simulink library "inp"  (R2021b)
settings: Solver=VariableStepAuto  StartTime=0.0  StopTime=10.0  RelTol=1e-3
undefined symbols (not defined in the file): C_TASK_5MS_S, FALSE, KINP_AcoreReadyToSlp_flg_ovrdflg, KINP_AcoreReadyToSlp_flg_ovrdval, KINP_AllowMovThd_OTA_enum_ovrdflg, KINP_AllowMovThd_OTA_enum_ovrdval, KINP_APSAngleTarget_Deg_ovrdflg, KINP_APSAngleTarget_Deg_ovrdval, KINP_APSDecReq_mps2_ovrdflg, KINP_APSDecReq_mps2_ovrdval, KINP_APSDecReqA_flg_ovrdflg, KINP_APSDecReqA_flg_ovrdval, KINP_APSDFLL_cm_ovrdflg, KINP_APSDFLL_cm_ovrdval, KINP_APSDFLR_cm_ovrdflg, KINP_APSDFLR_cm_ovrdval, KINP_APSDRLL_cm_ovrdflg, KINP_APSDRLL_cm_ovrdval, KINP_APSDRLR_cm_ovrdflg, KINP_APSDRLR_cm_ovrdval, KINP_APSExitCondition_enum_ovrdflg, KINP_APSExitCondition_enum_ovrdval, KINP_APSHWVer_enum_ovrdflg, KINP_APSHWVer_enum_ovrdval, KINP_APSProgressPCT_pct_ovrdflg, KINP_APSProgressPCT_pct_ovrdval, KINP_APSReq_enum_ovrdflg, KINP_APSReq_enum_ovrdval, KINP_APSRQDisplay_enum_ovrdflg, KINP_APSRQDisplay_enum_ovrdval, KINP_APSRqEPASCtrl_flg_ovrdflg, KINP_APSRqEPASCtrl_flg_ovrdval, KINP_APSShiftPosnReq_enum_ovrdval, KINP_APSShiftPosnReq_enum_ovrflg, KINP_APSSpeedCMD_kph_ovrdval, KINP_APSSpeedCMD_kph_ovrflg, KINP_APSStaSystem_enum_ovrdflg, KINP_APSStaSystem_enum_ovrdval, KINP_APSSWVer_enum_ovrdflg, KINP_APSSWVer_enum_ovrdval, KINP_APSVMCReqA_flg_ovrdval, KINP_APSVMCReqA_flg_ovrflg, KINP_APSVRqEPASCtrl_flg_ovrdflg, KINP_APSVRqEPASCtrl_flg_ovrdval, KINP_AuxBattVolmV_mV_ovrdflg, KINP_AuxBattVolmV_mV_ovrdval, KINP_CAASSta_enum_ovrdflg, KINP_CAASSta_enum_ovrdval, KINP_CAASVMCReqA_flg_ovrdval, KINP_CAASVMCReqA_flg_ovrflg, KINP_Chime_enum_ovrdflg, KINP_Chime_enum_ovrdval, KINP_ClearDTCcmd_flg_ovrdflg, KINP_ClearDTCcmd_flg_ovrdval, KINP_EvccAplusPwrUpReq_flg_ovrdflg, KINP_EvccAplusPwrUpReq_flg_ovrdval, KINP_LFID_raw_ovrdval, KINP_LFID_raw_ovrflg, KINP_LRID_raw_ovrdval, KINP_MemOffsetAccX_raw16_ovrdflg ... (+118)
libraries: FVT_lib x595, hcu_lib x1
(part 9 of 27)

== system inp/INP/CAN1/SignalCheck/EPAS2 ==
  BHAL_outputs : Inport
  inp_CanValid_bus : Inport  Port=2
  SASAngle : FVT_lib/inp/can_signal_template  SystemSampleTime=-1  VariantActivationTime=update diagram  Latency=0  AutoFrameSizeCalculation=off
      link override defval: Value=KINP_SASAngle_Deg_defval
      link override fftdec: Value=KINP_SASAngle_Deg_fftdec
      link override fftinc: Value=KINP_SASAngle_Deg_fftinc
      link override fftlim: Value=KINP_SASAngle_Deg_fftlim
      link override invalid: Value=KINP_SASAngle_Deg_invalid
      link override ovrdflg: Value=KINP_SASAngle_Deg_ovrdflg
      link override ovrdval: Value=KINP_SASAngle_Deg_ovrdval
      link override setvalid: Value=KINP_SASAngle_Deg_setvalid
      link override srvcflg: Value=KINP_SASAngle_Deg_srvcflg
      link override srvcval: Value=KINP_SASAngle_Deg_srvcval
  SASCAL : FVT_lib/inp/can_signal_template  SystemSampleTime=-1  VariantActivationTime=update diagram  Latency=0  AutoFrameSizeCalculation=off
      link override defval: Value=KINP_SASCAL_flg_defval
      link override fftdec: Value=KINP_SASCAL_flg_fftdec
      link override fftinc: Value=KINP_SASCAL_flg_fftinc
      link override fftlim: Value=KINP_SASCAL_flg_fftlim
      link override invalid: Value=KINP_SASCAL_flg_invalid
      link override ovrdflg: Value=KINP_SASCAL_flg_ovrdflg
      link override ovrdval: Value=KINP_SASCAL_flg_ovrdval
      link override setvalid: Value=KINP_SASCAL_flg_setvalid
      link override srvcflg: Value=KINP_SASCAL_flg_srvcflg
      link override srvcval: Value=KINP_SASCAL_flg_srvcval
  SASSpeed : FVT_lib/inp/can_signal_template  SystemSampleTime=-1  VariantActivationTime=update diagram  Latency=0  AutoFrameSizeCalculation=off
      link override defval: Value=KINP_SASSpeed_degps_defval
      link override fftdec: Value=KINP_SASSpeed_degps_fftdec
      link override fftinc: Value=KINP_SASSpeed_degps_fftinc
      link override fftlim: Value=KINP_SASSpeed_degps_fftlim
      link override invalid: Value=KINP_SASSpeed_degps_invalid
      link override ovrdflg: Value=KINP_SASSpeed_degps_ovrdflg
      link override ovrdval: Value=KINP_SASSpeed_degps_ovrdval
      link override setvalid: Value=KINP_SASSpeed_degps_setvalid
      link override srvcflg: Value=KINP_SASSpeed_degps_srvcflg
      link override srvcval: Value=KINP_SASSpeed_degps_srvcval
  SASSpeedValid : FVT_lib/inp/can_signal_template  SystemSampleTime=-1  VariantActivationTime=update diagram  Latency=0  AutoFrameSizeCalculation=off
      link override defval: Value=KINP_SASSpeedValid_flg_defval
      link override fftdec: Value=KINP_SASSpeedValid_flg_fftdec
      link override fftinc: Value=KINP_SASSpeedValid_flg_fftinc
      link override fftlim: Value=KINP_SASSpeedValid_flg_fftlim
      link override invalid: Value=KINP_SASSpeedValid_flg_invalid
      link override ovrdflg: Value=KINP_SASSpeedValid_flg_ovrdflg
      link override ovrdval: Value=KINP_SASSpeedValid_flg_ovrdval
      link override setvalid: Value=KINP_SASSpeedValid_flg_setvalid
      link override srvcflg: Value=KINP_SASSpeedValid_flg_srvcflg
      link override srvcval: Value=KINP_SASSpeedValid_flg_srvcval
  SASV : FVT_lib/inp/can_signal_template  SystemSampleTime=-1  VariantActivationTime=update diagram  Latency=0  AutoFrameSizeCalculation=off
      link override defval: Value=KINP_SASV_flg_defval
      link override fftdec: Value=KINP_SASV_flg_fftdec
      link override fftinc: Value=KINP_SASV_flg_fftinc
      link override fftlim: Value=KINP_SASV_flg_fftlim
      link override invalid: Value=KINP_SASV_flg_invalid
      link override ovrdflg: Value=KINP_SASV_flg_ovrdflg
      link override ovrdval: Value=KINP_SASV_flg_ovrdval
      link override setvalid: Value=KINP_SASV_flg_setvalid
      link override srvcflg: Value=KINP_SASV_flg_srvcflg
      link override srvcval: Value=KINP_SASV_flg_srvcval
  Terminator_{1..5} (5 alike) : Terminator
  True_VHAL_SASAngle_Deg : Constant  Value=TRUE  OutDataTypeStr=boolean
  True_VHAL_SASCAL_flg : Constant  Value=TRUE  OutDataTypeStr=boolean
  True_VHAL_SASSpeedValid_flg : Constant  Value=TRUE  OutDataTypeStr=boolean
  True_VHAL_SASSpeed_degps : Constant  Value=TRUE  OutDataTypeStr=boolean
  True_VHAL_SASV_flg : Constant  Value=TRUE  OutDataTypeStr=boolean
  slr1_{1..5} (5 alike) : BusSelector  OutputSignals=VINP_CANMsgValidEPAS2_flg
  slr_VHAL_SASAngle_Deg : BusSelector  OutputSignals=VHAL_SASAngle_Deg
  slr_VHAL_SASCAL_flg : BusSelector  OutputSignals=VHAL_SASCAL_flg
  slr_VHAL_SASSpeedValid_flg : BusSelector  OutputSignals=VHAL_SASSpeedValid_flg
  slr_VHAL_SASSpeed_degps : BusSelector  OutputSignals=VHAL_SASSpeed_degps
  slr_VHAL_SASV_flg : BusSelector  OutputSignals=VHAL_SASV_flg
  VINP_SASAngle_Deg : Outport
  VINP_SASCAL_flg : Outport  Port=2
  VINP_SASSpeed_degps : Outport  Port=3
  VINP_SASSpeedValid_flg : Outport  Port=4
  VINP_SASV_flg : Outport  Port=5
  wires:
  BHAL_outputs/1 -> [BHAL_outputs]
  inp_CanValid_bus/1 -> [inp_CanValid_bus]
  [BHAL_outputs] -> slr_VHAL_SASAngle_Deg/1
  slr_VHAL_SASAngle_Deg/1 -> SASAngle/1  "<VHAL_SASAngle_Deg>"
  True_VHAL_SASAngle_Deg/1 -> SASAngle/2
  [inp_CanValid_bus] -> slr1_1/1
  slr1_1/1 -> SASAngle/3  "<VINP_CANMsgValidEPAS2_flg>"
  SASAngle/1 -> VINP_SASAngle_Deg/1  "VINP_SASAngle_Deg"
  SASAngle/2 -> Terminator_1/1
  [BHAL_outputs] -> slr_VHAL_SASCAL_flg/1
  slr_VHAL_SASCAL_flg/1 -> SASCAL/1  "<VHAL_SASCAL_flg>"
  True_VHAL_SASCAL_flg/1 -> SASCAL/2
  [inp_CanValid_bus] -> slr1_2/1
  slr1_2/1 -> SASCAL/3  "<VINP_CANMsgValidEPAS2_flg>"
  SASCAL/1 -> VINP_SASCAL_flg/1  "VINP_SASCAL_flg"
  SASCAL/2 -> Terminator_2/1
  [BHAL_outputs] -> slr_VHAL_SASSpeed_degps/1
  slr_VHAL_SASSpeed_degps/1 -> SASSpeed/1  "<VHAL_SASSpeed_degps>"
  True_VHAL_SASSpeed_degps/1 -> SASSpeed/2
  [inp_CanValid_bus] -> slr1_3/1
  slr1_3/1 -> SASSpeed/3  "<VINP_CANMsgValidEPAS2_flg>"
  SASSpeed/1 -> VINP_SASSpeed_degps/1  "VINP_SASSpeed_degps"
  SASSpeed/2 -> Terminator_3/1
  [BHAL_outputs] -> slr_VHAL_SASSpeedValid_flg/1
  slr_VHAL_SASSpeedValid_flg/1 -> SASSpeedValid/1  "<VHAL_SASSpeedValid_flg>"
  True_VHAL_SASSpeedValid_flg/1 -> SASSpeedValid/2
  [inp_CanValid_bus] -> slr1_4/1
  slr1_4/1 -> SASSpeedValid/3  "<VINP_CANMsgValidEPAS2_flg>"
  SASSpeedValid/1 -> VINP_SASSpeedValid_flg/1  "VINP_SASSpeedValid_flg"
  SASSpeedValid/2 -> Terminator_4/1
  [BHAL_outputs] -> slr_VHAL_SASV_flg/1
  slr_VHAL_SASV_flg/1 -> SASV/1  "<VHAL_SASV_flg>"
  True_VHAL_SASV_flg/1 -> SASV/2
  [inp_CanValid_bus] -> slr1_5/1
  slr1_5/1 -> SASV/3  "<VINP_CANMsgValidEPAS2_flg>"
  SASV/1 -> VINP_SASV_flg/1  "VINP_SASV_flg"
  SASV/2 -> Terminator_5/1

== system inp/INP/CAN1/SignalCheck/EPB1 ==
  BHAL_outputs : Inport
  inp_CanValid_bus : Inport  Port=2
  DOASta : FVT_lib/inp/can_signal_template  SystemSampleTime=-1  VariantActivationTime=update diagram  Latency=0  AutoFrameSizeCalculation=off
      link override defval: Value=KINP_DOASta_flg_defval
      link override fftdec: Value=KINP_DOASta_flg_fftdec
      link override fftinc: Value=KINP_DOASta_flg_fftinc
      link override fftlim: Value=KINP_DOASta_flg_fftlim
      link override invalid: Value=KINP_DOASta_flg_invalid
      link override ovrdflg: Value=KINP_DOASta_flg_ovrdflg
      link override ovrdval: Value=KINP_DOASta_flg_ovrdval
      link override setvalid: Value=KINP_DOASta_flg_setvalid
      link override srvcflg: Value=KINP_DOASta_flg_srvcflg
      link override srvcval: Value=KINP_DOASta_flg_srvcval
  EPBCarWashMode : FVT_lib/inp/can_signal_template  SystemSampleTime=-1  VariantActivationTime=update diagram  Latency=0  AutoFrameSizeCalculation=off
      link override defval: Value=KINP_EPBCarWashMode_flg_defval
      link override fftdec: Value=KINP_EPBCarWashMode_flg_fftdec
      link override fftinc: Value=KINP_EPBCarWashMode_flg_fftinc
      link override fftlim: Value=KINP_EPBCarWashMode_flg_fftlim
      link override invalid: Value=KINP_EPBCarWashMode_flg_invalid
      link override ovrdflg: Value=KINP_EPBCarWashMode_flg_ovrdflg
      link override ovrdval: Value=KINP_EPBCarWashMode_flg_ovrdval
      link override setvalid: Value=KINP_EPBCarWashMode_flg_setvalid
      link override srvcflg: Value=KINP_EPBCarWashMode_flg_srvcflg
      link override srvcval: Value=KINP_EPBCarWashMode_flg_srvcval
  EPBErrSta : FVT_lib/inp/can_signal_template  SystemSampleTime=-1  VariantActivationTime=update diagram  Latency=0  AutoFrameSizeCalculation=off
      link override defval: Value=KINP_EPBErrSta_enum_defval
      link override fftdec: Value=KINP_EPBErrSta_enum_fftdec
      link override fftinc: Value=KINP_EPBErrSta_enum_fftinc
      link override fftlim: Value=KINP_EPBErrSta_enum_fftlim
      link override invalid: Value=KINP_EPBErrSta_enum_invalid
      link override ovrdflg: Value=KINP_EPBErrSta_enum_ovrdflg
      link override ovrdval: Value=KINP_EPBErrSta_enum_ovrdval
      link override setvalid: Value=KINP_EPBErrSta_enum_setvalid
      link override srvcflg: Value=KINP_EPBErrSta_enum_srvcflg
      link override srvcval: Value=KINP_EPBErrSta_enum_srvcval
  EPBExtApplyAvail : FVT_lib/inp/can_signal_template  SystemSampleTime=-1  VariantActivationTime=update diagram  Latency=0  AutoFrameSizeCalculation=off
      link override defval: Value=KINP_EPBExtApplyAvail_flg_defval
      link override fftdec: Value=KINP_EPBExtApplyAvail_flg_fftdec
      link override fftinc: Value=KINP_EPBExtApplyAvail_flg_fftinc
      link override fftlim: Value=KINP_EPBExtApplyAvail_flg_fftlim
      link override invalid: Value=KINP_EPBExtApplyAvail_flg_invalid
      link override ovrdflg: Value=KINP_EPBExtApplyAvail_flg_ovrdflg
      link override ovrdval: Value=KINP_EPBExtApplyAvail_flg_ovrdval
      link override setvalid: Value=KINP_EPBExtApplyAvail_flg_setvalid
      link override srvcflg: Value=KINP_EPBExtApplyAvail_flg_srvcflg
      link override srvcval: Value=KINP_EPBExtApplyAvail_flg_srvcval
  EPBExtReleaseAvail : FVT_lib/inp/can_signal_template  SystemSampleTime=-1  VariantActivationTime=update diagram  Latency=0  AutoFrameSizeCalculation=off
      link override defval: Value=KINP_EPBExtReleaseAvail_flg_defval
      link override fftdec: Value=KINP_EPBExtReleaseAvail_flg_fftdec
      link override fftinc: Value=KINP_EPBExtReleaseAvail_flg_fftinc
      link override fftlim: Value=KINP_EPBExtReleaseAvail_flg_fftlim
      link override invalid: Value=KINP_EPBExtReleaseAvail_flg_invalid
      link override ovrdflg: Value=KINP_EPBExtReleaseAvail_flg_ovrdflg
      link override ovrdval: Value=KINP_EPBExtReleaseAvail_flg_ovrdval
      link override setvalid: Value=KINP_EPBExtReleaseAvail_flg_setvalid
      link override srvcflg: Value=KINP_EPBExtReleaseAvail_flg_srvcflg
      link override srvcval: Value=KINP_EPBExtReleaseAvail_flg_srvcval
  EPBSta : FVT_lib/inp/can_signal_template  SystemSampleTime=-1  VariantActivationTime=update diagram  Latency=0  AutoFrameSizeCalculation=off
      link override defval: Value=KINP_EPBSta_enum_defval
      link override fftdec: Value=KINP_EPBSta_enum_fftdec
      link override fftinc: Value=KINP_EPBSta_enum_fftinc
      link override fftlim: Value=KINP_EPBSta_enum_fftlim
      link override invalid: Value=KINP_EPBSta_enum_invalid
      link override ovrdflg: Value=KINP_EPBSta_enum_ovrdflg
      link override ovrdval: Value=KINP_EPBSta_enum_ovrdval
      link override setvalid: Value=KINP_EPBSta_enum_setvalid
      link override srvcflg: Value=KINP_EPBSta_enum_srvcflg
      link override srvcval: Value=KINP_EPBSta_enum_srvcval
  Terminator_{1..6} (6 alike) : Terminator
  True_VHAL_DOASta_flg : Constant  Value=TRUE  OutDataTypeStr=boolean
  True_VHAL_EPBCarWashMode_flg : Constant  Value=TRUE  OutDataTypeStr=boolean
  True_VHAL_EPBErrSta_enum : Constant  Value=TRUE  OutDataTypeStr=boolean
  True_VHAL_EPBExtApplyAvail_flg : Constant  Value=TRUE  OutDataTypeStr=boolean
  True_VHAL_EPBExtReleaseAvail_flg : Constant  Value=TRUE  OutDataTypeStr=boolean
  True_VHAL_EPBSta_enum : Constant  Value=TRUE  OutDataTypeStr=boolean
  slr1_{1..6} (6 alike) : BusSelector  OutputSignals=VINP_CANMsgValidEPB1_flg
  slr_VHAL_DOASta_flg : BusSelector  OutputSignals=VHAL_DOASta_flg
  slr_VHAL_EPBCarWashMode_flg : BusSelector  OutputSignals=VHAL_EPBCarWashMode_flg
  slr_VHAL_EPBErrSta_enum : BusSelector  OutputSignals=VHAL_EPBErrSta_enum
  slr_VHAL_EPBExtApplyAvail_flg : BusSelector  OutputSignals=VHAL_EPBExtApplyAvail_flg
  slr_VHAL_EPBExtReleaseAvail_flg : BusSelector  OutputSignals=VHAL_EPBExtReleaseAvail_flg
  slr_VHAL_EPBSta_enum : BusSelector  OutputSignals=VHAL_EPBSta_enum
  VINP_DOASta_flg : Outport
  VINP_EPBCarWashMode_flg : Outport  Port=2
  VINP_EPBErrSta_enum : Outport  Port=3
  VINP_EPBExtApplyAvail_flg : Outport  Port=4
  VINP_EPBExtReleaseAvail_flg : Outport  Port=5
  VINP_EPBSta_enum : Outport  Port=6
  wires:
  BHAL_outputs/1 -> [BHAL_outputs]
  inp_CanValid_bus/1 -> [inp_CanValid_bus]
  [BHAL_outputs] -> slr_VHAL_DOASta_flg/1
  slr_VHAL_DOASta_flg/1 -> DOASta/1  "<VHAL_DOASta_flg>"
  True_VHAL_DOASta_flg/1 -> DOASta/2
  [inp_CanValid_bus] -> slr1_1/1
  slr1_1/1 -> DOASta/3  "<VINP_CANMsgValidEPB1_flg>"
  DOASta/1 -> VINP_DOASta_flg/1  "VINP_DOASta_flg"
  DOASta/2 -> Terminator_1/1
  [BHAL_outputs] -> slr_VHAL_EPBCarWashMode_flg/1
  slr_VHAL_EPBCarWashMode_flg/1 -> EPBCarWashMode/1  "<VHAL_EPBCarWashMode_flg>"
  True_VHAL_EPBCarWashMode_flg/1 -> EPBCarWashMode/2
  [inp_CanValid_bus] -> slr1_2/1
  slr1_2/1 -> EPBCarWashMode/3  "<VINP_CANMsgValidEPB1_flg>"
  EPBCarWashMode/1 -> VINP_EPBCarWashMode_flg/1  "VINP_EPBCarWashMode_flg"
  EPBCarWashMode/2 -> Terminator_2/1
  [BHAL_outputs] -> slr_VHAL_EPBErrSta_enum/1
  slr_VHAL_EPBErrSta_enum/1 -> EPBErrSta/1  "<VHAL_EPBErrSta_enum>"
  True_VHAL_EPBErrSta_enum/1 -> EPBErrSta/2
  [inp_CanValid_bus] -> slr1_3/1
  slr1_3/1 -> EPBErrSta/3  "<VINP_CANMsgValidEPB1_flg>"
  EPBErrSta/1 -> VINP_EPBErrSta_enum/1  "VINP_EPBErrSta_enum"
  EPBErrSta/2 -> Terminator_3/1
  [BHAL_outputs] -> slr_VHAL_EPBExtApplyAvail_flg/1
  slr_VHAL_EPBExtApplyAvail_flg/1 -> EPBExtApplyAvail/1  "<VHAL_EPBExtApplyAvail_flg>"
  True_VHAL_EPBExtApplyAvail_flg/1 -> EPBExtApplyAvail/2
  [inp_CanValid_bus] -> slr1_4/1
  slr1_4/1 -> EPBExtApplyAvail/3  "<VINP_CANMsgValidEPB1_flg>"
  EPBExtApplyAvail/1 -> VINP_EPBExtApplyAvail_flg/1  "VINP_EPBExtApplyAvail_flg"
  EPBExtApplyAvail/2 -> Terminator_4/1
  [BHAL_outputs] -> slr_VHAL_EPBExtReleaseAvail_flg/1
  slr_VHAL_EPBExtReleaseAvail_flg/1 -> EPBExtReleaseAvail/1  "<VHAL_EPBExtReleaseAvail_flg>"
  True_VHAL_EPBExtReleaseAvail_flg/1 -> EPBExtReleaseAvail/2
  [inp_CanValid_bus] -> slr1_5/1
  slr1_5/1 -> EPBExtReleaseAvail/3  "<VINP_CANMsgValidEPB1_flg>"
  EPBExtReleaseAvail/1 -> VINP_EPBExtReleaseAvail_flg/1  "VINP_EPBExtReleaseAvail_flg"
  EPBExtReleaseAvail/2 -> Terminator_5/1
  [BHAL_outputs] -> slr_VHAL_EPBSta_enum/1
  slr_VHAL_EPBSta_enum/1 -> EPBSta/1  "<VHAL_EPBSta_enum>"
  True_VHAL_EPBSta_enum/1 -> EPBSta/2
  [inp_CanValid_bus] -> slr1_6/1
  slr1_6/1 -> EPBSta/3  "<VINP_CANMsgValidEPB1_flg>"
  EPBSta/1 -> VINP_EPBSta_enum/1  "VINP_EPBSta_enum"
  EPBSta/2 -> Terminator_6/1

== system inp/INP/CAN1/SignalCheck/ESC1 ==
  BHAL_outputs : Inport
  inp_CanValid_bus : Inport  Port=2
  ESC1CS : FVT_lib/inp/can_signal_template  SystemSampleTime=-1  VariantActivationTime=update diagram  Latency=0  AutoFrameSizeCalculation=off
      link override defval: Value=KINP_ESC1CS_enum_defval
      link override fftdec: Value=KINP_ESC1CS_enum_fftdec
      link override fftinc: Value=KINP_ESC1CS_enum_fftinc
      link override fftlim: Value=KINP_ESC1CS_enum_fftlim
      link override invalid: Value=KINP_ESC1CS_enum_invalid
      link override ovrdflg: Value=KINP_ESC1CS_enum_ovrdflg
      link override ovrdval: Value=KINP_ESC1CS_enum_ovrdval
      link override setvalid: Value=KINP_ESC1CS_enum_setvalid
      link override srvcflg: Value=KINP_ESC1CS_enum_srvcflg
      link override srvcval: Value=KINP_ESC1CS_enum_srvcval
  ESC1CSErr : FVT_lib/inp/can_signal_template  SystemSampleTime=-1  VariantActivationTime=update diagram  Latency=0  AutoFrameSizeCalculation=off
      link override defval: Value=KINP_ESC1CSErr_flg_defval
      link override fftdec: Value=KINP_ESC1CSErr_flg_fftdec
      link override fftinc: Value=KINP_ESC1CSErr_flg_fftinc
      link override fftlim: Value=KINP_ESC1CSErr_flg_fftlim
      link override invalid: Value=KINP_ESC1CSErr_flg_invalid
      link override ovrdflg: Value=KINP_ESC1CSErr_flg_ovrdflg
      link override ovrdval: Value=KINP_ESC1CSErr_flg_ovrdval
      link override setvalid: Value=KINP_ESC1CSErr_flg_setvalid
      link override srvcflg: Value=KINP_ESC1CSErr_flg_srvcflg
      link override srvcval: Value=KINP_ESC1CSErr_flg_srvcval
  ESC1RC : FVT_lib/inp/can_signal_template  SystemSampleTime=-1  VariantActivationTime=update diagram  Latency=0  AutoFrameSizeCalculation=off
      link override defval: Value=KINP_ESC1RC_enum_defval
      link override fftdec: Value=KINP_ESC1RC_enum_fftdec
      link override fftinc: Value=KINP_ESC1RC_enum_fftinc
      link override fftlim: Value=KINP_ESC1RC_enum_fftlim
      link override invalid: Value=KINP_ESC1RC_enum_invalid
      link override ovrdflg: Value=KINP_ESC1RC_enum_ovrdflg
      link override ovrdval: Value=KINP_ESC1RC_enum_ovrdval
      link override setvalid: Value=KINP_ESC1RC_enum_setvalid
      link override srvcflg: Value=KINP_ESC1RC_enum_srvcflg
      link override srvcval: Value=KINP_ESC1RC_enum_srvcval
  ESC1RCErr : FVT_lib/inp/can_signal_template  SystemSampleTime=-1  VariantActivationTime=update diagram  Latency=0  AutoFrameSizeCalculation=off
      link override defval: Value=KINP_ESC1RCErr_flg_defval
      link override fftdec: Value=KINP_ESC1RCErr_flg_fftdec
      link override fftinc: Value=KINP_ESC1RCErr_flg_fftinc
      link override fftlim: Value=KINP_ESC1RCErr_flg_fftlim
      link override invalid: Value=KINP_ESC1RCErr_flg_invalid
      link override ovrdflg: Value=KINP_ESC1RCErr_flg_ovrdflg
      link override ovrdval: Value=KINP_ESC1RCErr_flg_ovrdval
      link override setvalid: Value=KINP_ESC1RCErr_flg_setvalid
      link override srvcflg: Value=KINP_ESC1RCErr_flg_srvcflg
      link override srvcval: Value=KINP_ESC1RCErr_flg_srvcval
  FrPTCSActive : FVT_lib/inp/can_signal_template  SystemSampleTime=-1  VariantActivationTime=update diagram  Latency=0  AutoFrameSizeCalculation=off
      link override defval: Value=KINP_FrPTCSActive_flg_defval
      link override fftdec: Value=KINP_FrPTCSActive_flg_fftdec
      link override fftinc: Value=KINP_FrPTCSActive_flg_fftinc
      link override fftlim: Value=KINP_FrPTCSActive_flg_fftlim
      link override invalid: Value=KINP_FrPTCSActive_flg_invalid
      link override ovrdflg: Value=KINP_FrPTCSActive_flg_ovrdflg
      link override ovrdval: Value=KINP_FrPTCSActive_flg_ovrdval
      link override setvalid: Value=KINP_FrPTCSActive_flg_setvalid
      link override srvcflg: Value=KINP_FrPTCSActive_flg_srvcflg
      link override srvcval: Value=KINP_FrPTCSActive_flg_srvcval
  FrntAxlTrqReqDrv : FVT_lib/inp/can_signal_template  SystemSampleTime=-1  VariantActivationTime=update diagram  Latency=0  AutoFrameSizeCalculation=off
      link override defval: Value=KINP_FrntAxlTrqReqDrv_Nm_defval
      link override fftdec: Value=KINP_FrntAxlTrqReqDrv_Nm_fftdec
      link override fftinc: Value=KINP_FrntAxlTrqReqDrv_Nm_fftinc
      link override fftlim: Value=KINP_FrntAxlTrqReqDrv_Nm_fftlim
      link override invalid: Value=KINP_FrntAxlTrqReqDrv_Nm_invalid
      link override ovrdflg: Value=KINP_FrntAxlTrqReqDrv_Nm_ovrdflg
      link override ovrdval: Value=KINP_FrntAxlTrqReqDrv_Nm_ovrdval
      link override setvalid: Value=KINP_FrntAxlTrqReqDrv_Nm_setvalid
      link override srvcflg: Value=KINP_FrntAxlTrqReqDrv_Nm_srvcflg
      link override srvcval: Value=KINP_FrntAxlTrqReqDrv_Nm_srvcval
  RearAxlTrqReqDrv : FVT_lib/inp/can_signal_template  SystemSampleTime=-1  VariantActivationTime=update diagram  Latency=0  AutoFrameSizeCalculation=off
      link override defval: Value=KINP_RearAxlTrqReqDrv_Nm_defval
      link override fftdec: Value=KINP_RearAxlTrqReqDrv_Nm_fftdec
      link override fftinc: Value=KINP_RearAxlTrqReqDrv_Nm_fftinc
      link override fftlim: Value=KINP_RearAxlTrqReqDrv_Nm_fftlim
      link override invalid: Value=KINP_RearAxlTrqReqDrv_Nm_invalid
      link override ovrdflg: Value=KINP_RearAxlTrqReqDrv_Nm_ovrdflg
      link override ovrdval: Value=KINP_RearAxlTrqReqDrv_Nm_ovrdval
      link override setvalid: Value=KINP_RearAxlTrqReqDrv_Nm_setvalid
      link override srvcflg: Value=KINP_RearAxlTrqReqDrv_Nm_srvcflg
      link override srvcval: Value=KINP_RearAxlTrqReqDrv_Nm_srvcval
  RrPTCSActive : FVT_lib/inp/can_signal_template  SystemSampleTime=-1  VariantActivationTime=update diagram  Latency=0  AutoFrameSizeCalculation=off
      link override defval: Value=KINP_RrPTCSActive_flg_defval
      link override fftdec: Value=KINP_RrPTCSActive_flg_fftdec
      link override fftinc: Value=KINP_RrPTCSActive_flg_fftinc
      link override fftlim: Value=KINP_RrPTCSActive_flg_fftlim
      link override invalid: Value=KINP_RrPTCSActive_flg_invalid
      link override ovrdflg: Value=KINP_RrPTCSActive_flg_ovrdflg
      link override ovrdval: Value=KINP_RrPTCSActive_flg_ovrdval
      link override setvalid: Value=KINP_RrPTCSActive_flg_setvalid
      link override srvcflg: Value=KINP_RrPTCSActive_flg_srvcflg
      link override srvcval: Value=KINP_RrPTCSActive_flg_srvcval
  Terminator_{1..9} (9 alike) : Terminator
  True_VHAL_ESC1CSErr_flg : Constant  Value=TRUE  OutDataTypeStr=boolean
  True_VHAL_ESC1CS_enum : Constant  Value=TRUE  OutDataTypeStr=boolean
  True_VHAL_ESC1RCErr_flg : Constant  Value=TRUE  OutDataTypeStr=boolean
  True_VHAL_ESC1RC_enum : Constant  Value=TRUE  OutDataTypeStr=boolean
  True_VHAL_FrPTCSActive_flg : Constant  Value=TRUE  OutDataTypeStr=boolean
  True_VHAL_FrntAxlTrqReqDrv_Nm : Constant  Value=TRUE  OutDataTypeStr=boolean
  True_VHAL_RearAxlTrqReqDrv_Nm : Constant  Value=TRUE  OutDataTypeStr=boolean
  True_VHAL_RrPTCSActive_flg : Constant  Value=TRUE  OutDataTypeStr=boolean
  True_VHAL_VehSpeed_kph : Constant  Value=TRUE  OutDataTypeStr=boolean
  VehSpeed : FVT_lib/inp/can_signal_template  SystemSampleTime=-1  VariantActivationTime=update diagram  Latency=0  AutoFrameSizeCalculation=off
      link override defval: Value=KINP_VehSpeed_kph_defval
      link override fftdec: Value=KINP_VehSpeed_kph_fftdec
      link override fftinc: Value=KINP_VehSpeed_kph_fftinc
      link override fftlim: Value=KINP_VehSpeed_kph_fftlim
      link override invalid: Value=KINP_VehSpeed_kph_invalid
      link override ovrdflg: Value=KINP_VehSpeed_kph_ovrdflg
      link override ovrdval: Value=KINP_VehSpeed_kph_ovrdval
      link override setvalid: Value=KINP_VehSpeed_kph_setvalid
      link override srvcflg: Value=KINP_VehSpeed_kph_srvcflg
      link override srvcval: Value=KINP_VehSpeed_kph_srvcval
  slr1_{1..9} (9 alike) : BusSelector  OutputSignals=VINP_CANMsgValidESC1_flg
  slr_VHAL_ESC1CSErr_flg : BusSelector  OutputSignals=VHAL_ESC1CSErr_flg
  slr_VHAL_ESC1CS_enum : BusSelector  OutputSignals=VHAL_ESC1CS_enum
  slr_VHAL_ESC1RCErr_flg : BusSelector  OutputSignals=VHAL_ESC1RCErr_flg
  slr_VHAL_ESC1RC_enum : BusSelector  OutputSignals=VHAL_ESC1RC_enum
  slr_VHAL_FrPTCSActive_flg : BusSelector  OutputSignals=VHAL_FrPTCSActive_flg
  slr_VHAL_FrntAxlTrqReqDrv_Nm : BusSelector  OutputSignals=VHAL_FrntAxlTrqReqDrv_Nm
  slr_VHAL_RearAxlTrqReqDrv_Nm : BusSelector  OutputSignals=VHAL_RearAxlTrqReqDrv_Nm
  slr_VHAL_RrPTCSActive_flg : BusSelector  OutputSignals=VHAL_RrPTCSActive_flg
  slr_VHAL_VehSpeed_kph : BusSelector  OutputSignals=VHAL_VehSpeed_kph
  VINP_ESC1CSErr_flg : Outport
  VINP_ESC1RCErr_flg : Outport  Port=2
  VINP_ESC1CS_enum : Outport  Port=3
  VINP_ESC1RC_enum : Outport  Port=4
  VINP_FrPTCSActive_flg : Outport  Port=5
  VINP_FrntAxlTrqReqDrv_Nm : Outport  Port=6
  VINP_RearAxlTrqReqDrv_Nm : Outport  Port=7
  VINP_RrPTCSActive_flg : Outport  Port=8
  VINP_VehSpeed_kph : Outport  Port=9
  wires:
  BHAL_outputs/1 -> [BHAL_outputs]
  inp_CanValid_bus/1 -> [inp_CanValid_bus]
  [BHAL_outputs] -> slr_VHAL_ESC1CSErr_flg/1
  slr_VHAL_ESC1CSErr_flg/1 -> ESC1CSErr/1  "<VHAL_ESC1CSErr_flg>"
  True_VHAL_ESC1CSErr_flg/1 -> ESC1CSErr/2
  [inp_CanValid_bus] -> slr1_1/1
  slr1_1/1 -> ESC1CSErr/3  "<VINP_CANMsgValidESC1_flg>"
  ESC1CSErr/1 -> VINP_ESC1CSErr_flg/1  "VINP_ESC1CSErr_flg"
  ESC1CSErr/2 -> Terminator_1/1
  [BHAL_outputs] -> slr_VHAL_ESC1RCErr_flg/1
  slr_VHAL_ESC1RCErr_flg/1 -> ESC1RCErr/1  "<VHAL_ESC1RCErr_flg>"
  True_VHAL_ESC1RCErr_flg/1 -> ESC1RCErr/2
  [inp_CanValid_bus] -> slr1_2/1
  slr1_2/1 -> ESC1RCErr/3  "<VINP_CANMsgValidESC1_flg>"
  ESC1RCErr/1 -> VINP_ESC1RCErr_flg/1  "VINP_ESC1RCErr_flg"
  ESC1RCErr/2 -> Terminator_2/1
  [BHAL_outputs] -> slr_VHAL_ESC1CS_enum/1
  slr_VHAL_ESC1CS_enum/1 -> ESC1CS/1  "<VHAL_ESC1CS_enum>"
  True_VHAL_ESC1CS_enum/1 -> ESC1CS/2
  [inp_CanValid_bus] -> slr1_3/1
  slr1_3/1 -> ESC1CS/3  "<VINP_CANMsgValidESC1_flg>"
  ESC1CS/1 -> VINP_ESC1CS_enum/1  "VINP_ESC1CS_enum"
  ESC1CS/2 -> Terminator_3/1
  [BHAL_outputs] -> slr_VHAL_ESC1RC_enum/1
  slr_VHAL_ESC1RC_enum/1 -> ESC1RC/1  "<VHAL_ESC1RC_enum>"
  True_VHAL_ESC1RC_enum/1 -> ESC1RC/2
  [inp_CanValid_bus] -> slr1_4/1
  slr1_4/1 -> ESC1RC/3  "<VINP_CANMsgValidESC1_flg>"
  ESC1RC/1 -> VINP_ESC1RC_enum/1  "VINP_ESC1RC_enum"
  ESC1RC/2 -> Terminator_4/1
  [BHAL_outputs] -> slr_VHAL_FrPTCSActive_flg/1
  slr_VHAL_FrPTCSActive_flg/1 -> FrPTCSActive/1  "<VHAL_FrPTCSActive_flg>"
  True_VHAL_FrPTCSActive_flg/1 -> FrPTCSActive/2
  [inp_CanValid_bus] -> slr1_5/1
  slr1_5/1 -> FrPTCSActive/3  "<VINP_CANMsgValidESC1_flg>"
  FrPTCSActive/1 -> VINP_FrPTCSActive_flg/1  "VINP_FrPTCSActive_flg"
  FrPTCSActive/2 -> Terminator_5/1
  [BHAL_outputs] -> slr_VHAL_FrntAxlTrqReqDrv_Nm/1
  slr_VHAL_FrntAxlTrqReqDrv_Nm/1 -> FrntAxlTrqReqDrv/1  "<VHAL_FrntAxlTrqReqDrv_Nm>"
  True_VHAL_FrntAxlTrqReqDrv_Nm/1 -> FrntAxlTrqReqDrv/2
  [inp_CanValid_bus] -> slr1_6/1
  slr1_6/1 -> FrntAxlTrqReqDrv/3  "<VINP_CANMsgValidESC1_flg>"
  FrntAxlTrqReqDrv/1 -> VINP_FrntAxlTrqReqDrv_Nm/1  "VINP_FrntAxlTrqReqDrv_Nm"
  FrntAxlTrqReqDrv/2 -> Terminator_6/1
  [BHAL_outputs] -> slr_VHAL_RearAxlTrqReqDrv_Nm/1
  slr_VHAL_RearAxlTrqReqDrv_Nm/1 -> RearAxlTrqReqDrv/1  "<VHAL_RearAxlTrqReqDrv_Nm>"
  True_VHAL_RearAxlTrqReqDrv_Nm/1 -> RearAxlTrqReqDrv/2
  [inp_CanValid_bus] -> slr1_7/1
  slr1_7/1 -> RearAxlTrqReqDrv/3  "<VINP_CANMsgValidESC1_flg>"
  RearAxlTrqReqDrv/1 -> VINP_RearAxlTrqReqDrv_Nm/1  "VINP_RearAxlTrqReqDrv_Nm"
  RearAxlTrqReqDrv/2 -> Terminator_7/1
  [BHAL_outputs] -> slr_VHAL_RrPTCSActive_flg/1
  slr_VHAL_RrPTCSActive_flg/1 -> RrPTCSActive/1  "<VHAL_RrPTCSActive_flg>"
  True_VHAL_RrPTCSActive_flg/1 -> RrPTCSActive/2
  [inp_CanValid_bus] -> slr1_8/1
  slr1_8/1 -> RrPTCSActive/3  "<VINP_CANMsgValidESC1_flg>"
  RrPTCSActive/1 -> VINP_RrPTCSActive_flg/1  "VINP_RrPTCSActive_flg"
  RrPTCSActive/2 -> Terminator_8/1
  [BHAL_outputs] -> slr_VHAL_VehSpeed_kph/1
  slr_VHAL_VehSpeed_kph/1 -> VehSpeed/1  "<VHAL_VehSpeed_kph>"
  True_VHAL_VehSpeed_kph/1 -> VehSpeed/2
  [inp_CanValid_bus] -> slr1_9/1
  slr1_9/1 -> VehSpeed/3  "<VINP_CANMsgValidESC1_flg>"
  VehSpeed/1 -> VINP_VehSpeed_kph/1  "VINP_VehSpeed_kph"
  VehSpeed/2 -> Terminator_9/1

== system inp/INP/CAN1/SignalCheck/ESC2 ==
  BHAL_outputs : Inport
  inp_CanValid_bus : Inport  Port=2
  LFPulseCount : FVT_lib/inp/can_signal_template  SystemSampleTime=-1  VariantActivationTime=update diagram  Latency=0  AutoFrameSizeCalculation=off
      link override defval: Value=KINP_LFPulseCount_enum_defval
      link override fftdec: Value=KINP_LFPulseCount_enum_fftdec
      link override fftinc: Value=KINP_LFPulseCount_enum_fftinc
      link override fftlim: Value=KINP_LFPulseCount_enum_fftlim
      link override invalid: Value=KINP_LFPulseCount_enum_invalid
      link override ovrdflg: Value=KINP_LFPulseCount_enum_ovrdflg
      link override ovrdval: Value=KINP_LFPulseCount_enum_ovrdval
      link override setvalid: Value=KINP_LFPulseCount_enum_setvalid
      link override srvcflg: Value=KINP_LFPulseCount_enum_srvcflg
      link override srvcval: Value=KINP_LFPulseCount_enum_srvcval
  LFPulseCountV : FVT_lib/inp/can_signal_template  SystemSampleTime=-1  VariantActivationTime=update diagram  Latency=0  AutoFrameSizeCalculation=off
      link override defval: Value=KINP_LFPulseCountV_flg_defval
      link override fftdec: Value=KINP_LFPulseCountV_flg_fftdec
      link override fftinc: Value=KINP_LFPulseCountV_flg_fftinc
      link override fftlim: Value=KINP_LFPulseCountV_flg_fftlim
      link override invalid: Value=KINP_LFPulseCountV_flg_invalid
      link override ovrdflg: Value=KINP_LFPulseCountV_flg_ovrdflg
      link override ovrdval: Value=KINP_LFPulseCountV_flg_ovrdval
      link override setvalid: Value=KINP_LFPulseCountV_flg_setvalid
      link override srvcflg: Value=KINP_LFPulseCountV_flg_srvcflg
      link override srvcval: Value=KINP_LFPulseCountV_flg_srvcval
  LFRawWhlSpeed : FVT_lib/inp/can_signal_template  SystemSampleTime=-1  VariantActivationTime=update diagram  Latency=0  AutoFrameSizeCalculation=off
      link override defval: Value=KINP_LFRawWhlSpeed_kph_defval
      link override fftdec: Value=KINP_LFRawWhlSpeed_kph_fftdec
      link override fftinc: Value=KINP_LFRawWhlSpeed_kph_fftinc
      link override fftlim: Value=KINP_LFRawWhlSpeed_kph_fftlim
      link override invalid: Value=KINP_LFRawWhlSpeed_kph_invalid
      link override ovrdflg: Value=KINP_LFRawWhlSpeed_kph_ovrdflg
      link override ovrdval: Value=KINP_LFRawWhlSpeed_kph_ovrdval
      link override setvalid: Value=KINP_LFRawWhlSpeed_kph_setvalid
      link override srvcflg: Value=KINP_LFRawWhlSpeed_kph_srvcflg
      link override srvcval: Value=KINP_LFRawWhlSpeed_kph_srvcval
  LFRawWhlSpeedV : FVT_lib/inp/can_signal_template  SystemSampleTime=-1  VariantActivationTime=update diagram  Latency=0  AutoFrameSizeCalculation=off
      link override defval: Value=KINP_LFRawWhlSpeedV_flg_defval
      link override fftdec: Value=KINP_LFRawWhlSpeedV_flg_fftdec
      link override fftinc: Value=KINP_LFRawWhlSpeedV_flg_fftinc
      link override fftlim: Value=KINP_LFRawWhlSpeedV_flg_fftlim
      link override invalid: Value=KINP_LFRawWhlSpeedV_flg_invalid
      link override ovrdflg: Value=KINP_LFRawWhlSpeedV_flg_ovrdflg
      link override ovrdval: Value=KINP_LFRawWhlSpeedV_flg_ovrdval
      link override setvalid: Value=KINP_LFRawWhlSpeedV_flg_setvalid
      link override srvcflg: Value=KINP_LFRawWhlSpeedV_flg_srvcflg
      link override srvcval: Value=KINP_LFRawWhlSpeedV_flg_srvcval
  LFWhlRotDir : FVT_lib/inp/can_signal_template  SystemSampleTime=-1  VariantActivationTime=update diagram  Latency=0  AutoFrameSizeCalculation=off
      link override defval: Value=KINP_LFWhlRotDir_enum_defval
      link override fftdec: Value=KINP_LFWhlRotDir_enum_fftdec
      link override fftinc: Value=KINP_LFWhlRotDir_enum_fftinc
      link override fftlim: Value=KINP_LFWhlRotDir_enum_fftlim
      link override invalid: Value=KINP_LFWhlRotDir_enum_invalid
      link override ovrdflg: Value=KINP_LFWhlRotDir_enum_ovrdflg
      link override ovrdval: Value=KINP_LFWhlRotDir_enum_ovrdval
      link override setvalid: Value=KINP_LFWhlRotDir_enum_setvalid
      link override srvcflg: Value=KINP_LFWhlRotDir_enum_srvcflg
      link override srvcval: Value=KINP_LFWhlRotDir_enum_srvcval
  RFPulseCount : FVT_lib/inp/can_signal_template  SystemSampleTime=-1  VariantActivationTime=update diagram  Latency=0  AutoFrameSizeCalculation=off
      link override defval: Value=KINP_RFPulseCount_enum_defval
      link override fftdec: Value=KINP_RFPulseCount_enum_fftdec
      link override fftinc: Value=KINP_RFPulseCount_enum_fftinc
      link override fftlim: Value=KINP_RFPulseCount_enum_fftlim
      link override invalid: Value=KINP_RFPulseCount_enum_invalid
      link override ovrdflg: Value=KINP_RFPulseCount_enum_ovrdflg
      link override ovrdval: Value=KINP_RFPulseCount_enum_ovrdval
      link override setvalid: Value=KINP_RFPulseCount_enum_setvalid
      link override srvcflg: Value=KINP_RFPulseCount_enum_srvcflg
      link override srvcval: Value=KINP_RFPulseCount_enum_srvcval
  RFPulseCountV : FVT_lib/inp/can_signal_template  SystemSampleTime=-1  VariantActivationTime=update diagram  Latency=0  AutoFrameSizeCalculation=off
      link override defval: Value=KINP_RFPulseCountV_flg_defval
      link override fftdec: Value=KINP_RFPulseCountV_flg_fftdec
      link override fftinc: Value=KINP_RFPulseCountV_flg_fftinc
      link override fftlim: Value=KINP_RFPulseCountV_flg_fftlim
      link override invalid: Value=KINP_RFPulseCountV_flg_invalid
      link override ovrdflg: Value=KINP_RFPulseCountV_flg_ovrdflg
      link override ovrdval: Value=KINP_RFPulseCountV_flg_ovrdval
      link override setvalid: Value=KINP_RFPulseCountV_flg_setvalid
      link override srvcflg: Value=KINP_RFPulseCountV_flg_srvcflg
      link override srvcval: Value=KINP_RFPulseCountV_flg_srvcval
  RFRawWhlSpeed : FVT_lib/inp/can_signal_template  SystemSampleTime=-1  VariantActivationTime=update diagram  Latency=0  AutoFrameSizeCalculation=off
      link override defval: Value=KINP_RFRawWhlSpeed_kph_defval
      link override fftdec: Value=KINP_RFRawWhlSpeed_kph_fftdec
      link override fftinc: Value=KINP_RFRawWhlSpeed_kph_fftinc
      link override fftlim: Value=KINP_RFRawWhlSpeed_kph_fftlim
      link override invalid: Value=KINP_RFRawWhlSpeed_kph_invalid
      link override ovrdflg: Value=KINP_RFRawWhlSpeed_kph_ovrdflg
      link override ovrdval: Value=KINP_RFRawWhlSpeed_kph_ovrdval
      link override setvalid: Value=KINP_RFRawWhlSpeed_kph_setvalid
      link override srvcflg: Value=KINP_RFRawWhlSpeed_kph_srvcflg
      link override srvcval: Value=KINP_RFRawWhlSpeed_kph_srvcval
  RFRawWhlSpeedV : FVT_lib/inp/can_signal_template  SystemSampleTime=-1  VariantActivationTime=update diagram  Latency=0  AutoFrameSizeCalculation=off
      link override defval: Value=KINP_RFRawWhlSpeedV_flg_defval
      link override fftdec: Value=KINP_RFRawWhlSpeedV_flg_fftdec
      link override fftinc: Value=KINP_RFRawWhlSpeedV_flg_fftinc
      link override fftlim: Value=KINP_RFRawWhlSpeedV_flg_fftlim
      link override invalid: Value=KINP_RFRawWhlSpeedV_flg_invalid
      link override ovrdflg: Value=KINP_RFRawWhlSpeedV_flg_ovrdflg
      link override ovrdval: Value=KINP_RFRawWhlSpeedV_flg_ovrdval
      link override setvalid: Value=KINP_RFRawWhlSpeedV_flg_setvalid
      link override srvcflg: Value=KINP_RFRawWhlSpeedV_flg_srvcflg
      link override srvcval: Value=KINP_RFRawWhlSpeedV_flg_srvcval
  RFWhlRotDir : FVT_lib/inp/can_signal_template  SystemSampleTime=-1  VariantActivationTime=update diagram  Latency=0  AutoFrameSizeCalculation=off
      link override defval: Value=KINP_RFWhlRotDir_enum_defval
      link override fftdec: Value=KINP_RFWhlRotDir_enum_fftdec
      link override fftinc: Value=KINP_RFWhlRotDir_enum_fftinc
      link override fftlim: Value=KINP_RFWhlRotDir_enum_fftlim
      link override invalid: Value=KINP_RFWhlRotDir_enum_invalid
      link override ovrdflg: Value=KINP_RFWhlRotDir_enum_ovrdflg
      link override ovrdval: Value=KINP_RFWhlRotDir_enum_ovrdval
      link override setvalid: Value=KINP_RFWhlRotDir_enum_setvalid
      link override srvcflg: Value=KINP_RFWhlRotDir_enum_srvcflg
      link override srvcval: Value=KINP_RFWhlRotDir_enum_srvcval
  Terminator_{1..10} (10 alike) : Terminator
  True_VHAL_LFPulseCountV_flg : Constant  Value=TRUE  OutDataTypeStr=boolean
  True_VHAL_LFPulseCount_enum : Constant  Value=TRUE  OutDataTypeStr=boolean
  True_VHAL_LFRawWhlSpeedV_flg : Constant  Value=TRUE  OutDataTypeStr=boolean
  True_VHAL_LFRawWhlSpeed_kph : Constant  Value=TRUE  OutDataTypeStr=boolean
  True_VHAL_LFWhlRotDir_enum : Constant  Value=TRUE  OutDataTypeStr=boolean
  True_VHAL_RFPulseCountV_flg : Constant  Value=TRUE  OutDataTypeStr=boolean
  True_VHAL_RFPulseCount_enum : Constant  Value=TRUE  OutDataTypeStr=boolean
  True_VHAL_RFRawWhlSpeedV_flg : Constant  Value=TRUE  OutDataTypeStr=boolean
  True_VHAL_RFRawWhlSpeed_kph : Constant  Value=TRUE  OutDataTypeStr=boolean
  True_VHAL_RFWhlRotDir_enum : Constant  Value=TRUE  OutDataTypeStr=boolean
  slr1_{1..10} (10 alike) : BusSelector  OutputSignals=VINP_CANMsgValidESC2_flg
  slr_VHAL_LFPulseCountV_flg : BusSelector  OutputSignals=VHAL_LFPulseCountV_flg
  slr_VHAL_LFPulseCount_enum : BusSelector  OutputSignals=VHAL_LFPulseCount_enum
  slr_VHAL_LFRawWhlSpeedV_flg : BusSelector  OutputSignals=VHAL_LFRawWhlSpeedV_flg
  slr_VHAL_LFRawWhlSpeed_kph : BusSelector  OutputSignals=VHAL_LFRawWhlSpeed_kph
  slr_VHAL_LFWhlRotDir_enum : BusSelector  OutputSignals=VHAL_LFWhlRotDir_enum
  slr_VHAL_RFPulseCountV_flg : BusSelector  OutputSignals=VHAL_RFPulseCountV_flg
  slr_VHAL_RFPulseCount_enum : BusSelector  OutputSignals=VHAL_RFPulseCount_enum
  slr_VHAL_RFRawWhlSpeedV_flg : BusSelector  OutputSignals=VHAL_RFRawWhlSpeedV_flg
  slr_VHAL_RFRawWhlSpeed_kph : BusSelector  OutputSignals=VHAL_RFRawWhlSpeed_kph
  slr_VHAL_RFWhlRotDir_enum : BusSelector  OutputSignals=VHAL_RFWhlRotDir_enum
  VINP_LFPulseCount_enum : Outport
  VINP_LFPulseCountV_flg : Outport  Port=2
  VINP_LFRawWhlSpeed_kph : Outport  Port=3
  VINP_LFRawWhlSpeedV_flg : Outport  Port=4
  VINP_LFWhlRotDir_enum : Outport  Port=5
  VINP_RFPulseCount_enum : Outport  Port=6
  VINP_RFPulseCountV_flg : Outport  Port=7
  VINP_RFRawWhlSpeed_kph : Outport  Port=8
  VINP_RFRawWhlSpeedV_flg : Outport  Port=9
  VINP_RFWhlRotDir_enum : Outport  Port=10
  wires:
  BHAL_outputs/1 -> [BHAL_outputs]
  inp_CanValid_bus/1 -> [inp_CanValid_bus]
  [BHAL_outputs] -> slr_VHAL_LFPulseCount_enum/1
  slr_VHAL_LFPulseCount_enum/1 -> LFPulseCount/1  "<VHAL_LFPulseCount_enum>"
  True_VHAL_LFPulseCount_enum/1 -> LFPulseCount/2
  [inp_CanValid_bus] -> slr1_1/1
  slr1_1/1 -> LFPulseCount/3  "<VINP_CANMsgValidESC2_flg>"
  LFPulseCount/1 -> VINP_LFPulseCount_enum/1  "VINP_LFPulseCount_enum"
  LFPulseCount/2 -> Terminator_1/1
  [BHAL_outputs] -> slr_VHAL_LFPulseCountV_flg/1
  slr_VHAL_LFPulseCountV_flg/1 -> LFPulseCountV/1  "<VHAL_LFPulseCountV_flg>"
  True_VHAL_LFPulseCountV_flg/1 -> LFPulseCountV/2
  [inp_CanValid_bus] -> slr1_2/1
  slr1_2/1 -> LFPulseCountV/3  "<VINP_CANMsgValidESC2_flg>"
  LFPulseCountV/1 -> VINP_LFPulseCountV_flg/1  "VINP_LFPulseCountV_flg"
  LFPulseCountV/2 -> Terminator_2/1
  [BHAL_outputs] -> slr_VHAL_LFRawWhlSpeed_kph/1
  slr_VHAL_LFRawWhlSpeed_kph/1 -> LFRawWhlSpeed/1  "<VHAL_LFRawWhlSpeed_kph>"
  True_VHAL_LFRawWhlSpeed_kph/1 -> LFRawWhlSpeed/2
  [inp_CanValid_bus] -> slr1_3/1
  slr1_3/1 -> LFRawWhlSpeed/3  "<VINP_CANMsgValidESC2_flg>"
  LFRawWhlSpeed/1 -> VINP_LFRawWhlSpeed_kph/1  "VINP_LFRawWhlSpeed_kph"
  LFRawWhlSpeed/2 -> Terminator_3/1
  [BHAL_outputs] -> slr_VHAL_LFRawWhlSpeedV_flg/1
  slr_VHAL_LFRawWhlSpeedV_flg/1 -> LFRawWhlSpeedV/1  "<VHAL_LFRawWhlSpeedV_flg>"
  True_VHAL_LFRawWhlSpeedV_flg/1 -> LFRawWhlSpeedV/2
  [inp_CanValid_bus] -> slr1_4/1
  slr1_4/1 -> LFRawWhlSpeedV/3  "<VINP_CANMsgValidESC2_flg>"
  LFRawWhlSpeedV/1 -> VINP_LFRawWhlSpeedV_flg/1  "VINP_LFRawWhlSpeedV_flg"
  LFRawWhlSpeedV/2 -> Terminator_4/1
  [BHAL_outputs] -> slr_VHAL_LFWhlRotDir_enum/1
  slr_VHAL_LFWhlRotDir_enum/1 -> LFWhlRotDir/1  "<VHAL_LFWhlRotDir_enum>"
  True_VHAL_LFWhlRotDir_enum/1 -> LFWhlRotDir/2
  [inp_CanValid_bus] -> slr1_5/1
  slr1_5/1 -> LFWhlRotDir/3  "<VINP_CANMsgValidESC2_flg>"
  LFWhlRotDir/1 -> VINP_LFWhlRotDir_enum/1  "VINP_LFWhlRotDir_enum"
  LFWhlRotDir/2 -> Terminator_5/1
  [BHAL_outputs] -> slr_VHAL_RFPulseCount_enum/1
  slr_VHAL_RFPulseCount_enum/1 -> RFPulseCount/1  "<VHAL_RFPulseCount_enum>"
  True_VHAL_RFPulseCount_enum/1 -> RFPulseCount/2
  [inp_CanValid_bus] -> slr1_6/1
  slr1_6/1 -> RFPulseCount/3  "<VINP_CANMsgValidESC2_flg>"
  RFPulseCount/1 -> VINP_RFPulseCount_enum/1  "VINP_RFPulseCount_enum"
  RFPulseCount/2 -> Terminator_6/1
  [BHAL_outputs] -> slr_VHAL_RFPulseCountV_flg/1
  slr_VHAL_RFPulseCountV_flg/1 -> RFPulseCountV/1  "<VHAL_RFPulseCountV_flg>"
  True_VHAL_RFPulseCountV_flg/1 -> RFPulseCountV/2
  [inp_CanValid_bus] -> slr1_7/1
  slr1_7/1 -> RFPulseCountV/3  "<VINP_CANMsgValidESC2_flg>"
  RFPulseCountV/1 -> VINP_RFPulseCountV_flg/1  "VINP_RFPulseCountV_flg"
  RFPulseCountV/2 -> Terminator_7/1
  [BHAL_outputs] -> slr_VHAL_RFRawWhlSpeed_kph/1
  slr_VHAL_RFRawWhlSpeed_kph/1 -> RFRawWhlSpeed/1  "<VHAL_RFRawWhlSpeed_kph>"
  True_VHAL_RFRawWhlSpeed_kph/1 -> RFRawWhlSpeed/2
  [inp_CanValid_bus] -> slr1_8/1
  slr1_8/1 -> RFRawWhlSpeed/3  "<VINP_CANMsgValidESC2_flg>"
  RFRawWhlSpeed/1 -> VINP_RFRawWhlSpeed_kph/1  "VINP_RFRawWhlSpeed_kph"
  RFRawWhlSpeed/2 -> Terminator_8/1
  [BHAL_outputs] -> slr_VHAL_RFRawWhlSpeedV_flg/1
  slr_VHAL_RFRawWhlSpeedV_flg/1 -> RFRawWhlSpeedV/1  "<VHAL_RFRawWhlSpeedV_flg>"
  True_VHAL_RFRawWhlSpeedV_flg/1 -> RFRawWhlSpeedV/2
  [inp_CanValid_bus] -> slr1_9/1
  slr1_9/1 -> RFRawWhlSpeedV/3  "<VINP_CANMsgValidESC2_flg>"
  RFRawWhlSpeedV/1 -> VINP_RFRawWhlSpeedV_flg/1  "VINP_RFRawWhlSpeedV_flg"
  RFRawWhlSpeedV/2 -> Terminator_9/1
  [BHAL_outputs] -> slr_VHAL_RFWhlRotDir_enum/1
  slr_VHAL_RFWhlRotDir_enum/1 -> RFWhlRotDir/1  "<VHAL_RFWhlRotDir_enum>"
  True_VHAL_RFWhlRotDir_enum/1 -> RFWhlRotDir/2
  [inp_CanValid_bus] -> slr1_10/1
  slr1_10/1 -> RFWhlRotDir/3  "<VINP_CANMsgValidESC2_flg>"
  RFWhlRotDir/1 -> VINP_RFWhlRotDir_enum/1  "VINP_RFWhlRotDir_enum"
  RFWhlRotDir/2 -> Terminator_10/1
